simulink model "surrogate_block"  (R2025a)
settings: Solver=FixedStepDiscrete  StartTime=0.0  StopTime=1.0  FixedStep=1/2000  RelTol=1e-3
settings Model: Creator=yk  LastModifiedBy=yk

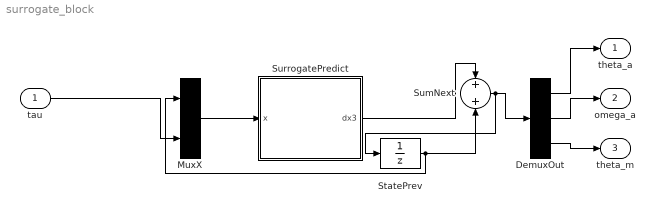
== system surrogate_block ==
  tau : Inport
  DemuxOut : Demux  Outputs=3
  MuxX : Mux  Inputs=2
  StatePrev : UnitDelay  InitialCondition=[0;0;0]  SampleTime=1/2000  HasFrameUpgradeWarning=on
  SumNext : Sum
  SurrogatePredict : MATLAB Function  TreatAsAtomicUnit=on
  theta_a : Outport
  omega_a : Outport  Port=2
  theta_m : Outport  Port=3
  wires:
  StatePrev/1 -> MuxX/1, SumNext/2
  tau/1 -> MuxX/2
  MuxX/1 -> SurrogatePredict/1(x)
  SurrogatePredict/1(dx3) -> SumNext/1
  SumNext/1 -> DemuxOut/1, StatePrev/1
  DemuxOut/1 -> theta_a/1
  DemuxOut/2 -> omega_a/1
  DemuxOut/3 -> theta_m/1

== matlab function surrogate_block/SurrogatePredict ==
  data: x input; dx3 output
function dx3 = surrogate_predict(x)
%#codegen
    dtheta_a = surrogate_sub_theta_a(x);
    domega_a = surrogate_sub_omega_a(x);
    dtheta_m = surrogate_sub_theta_m(x);
    dx3 = [dtheta_a; domega_a; dtheta_m];
end
